simulink library "bipedlib"  (Simulink 6.1)
values from neighbouring files (symbols this model uses):
  D = [Db1, Db2, Db3, Db4 ... (first row only)    [pdparams.m]
  g = 9.81    [bipedparams.m]
  initstate =     [initstate.mat]
  l1 = 0.5    [bipedparams.m]    (also in pdparams.m = robot.l(2))
  l2 = 0.5    [bipedparams.m]    (also in pdparams.m = robot.l(3))
  P = [Pb1, Pb2, Pb3, Pb4 ... (first row only)    [pdparams.m]
  r0 = l0/2    (= 0.4)    [bipedparams.m]    (also in pdparams.m = robot.r(1))
  ref = [0.04, 0.3261, 0.0314, 0.2199]'    [pdparams.m]
  st = 0.005    [bipedparams.m]    (also in pdparams.m)
undefined symbols (not defined in the file or in its folder): dataprop, groundp, initswitch, knees, robot
libraries: bipedlib x11, simulink x6, crclib x1
(part 1 of 2)
settings Model: LastModifiedBy=Olli Haavisto

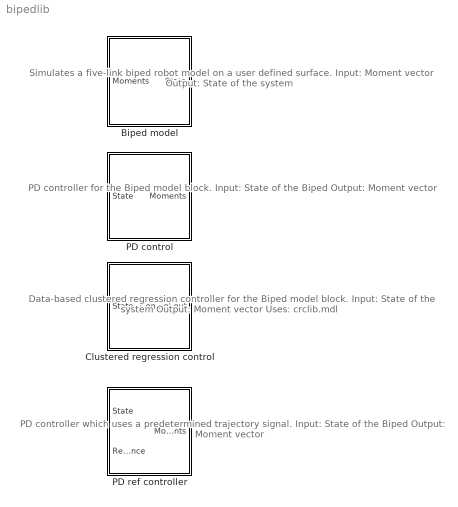
== system bipedlib ==
  note: Simulates a five-link biped robot model
      | on a user defined surface.
      | Input: Moment vector
      | Output: State of the system
  note: PD controller for the Biped model block.
      | Input: State of the Biped
      | Output: Moment vector
  note: Data-based clustered regression controller
      | for the Biped model block.
      | Input: State of the system
      | Output: Moment vector
      | Uses: crclib.mdl
  note: PD controller which uses a predetermined
      | trajectory signal.
      | Input: State of the Biped
      | Output: Moment vector
  Biped model : Subsystem  mask(Biped model){robot=robot, initstate=initstate, knees=knees, groundp=groundp, g=g, st=st}
      mask prompts: robot "Robot dimensions:"; initstate "Robot initial state:"; knees "Knee angle limiter parameters:"; groundp "Ground properties:"; g "Acceleration of gravity:"; st "Sample time:"
      mask help: The Biped model block simulates a 5-link biped walking robot on a user defined surface. The input is the moment vector and the output the state vector of the system.
      mask init:
      | % robot link lengths
      | l0 = robot.l(1); % torso
      | l1 = robot.l(2); % thigh
      | l2 = robot.l(3); % shank
      | % mass center locations
      | r0 = robot.r(1); % torso (from hip)
      | r1 = robot.r(2); % thigh (from hip)
      | r2 = robot.r(3); % shank (from knee)
      | % masses
      | m0 = robot.m(1); % torso
      | m1 = robot.m(2); % thigh
      | m2 = robot.m(3); % shank
      | % link inertias
      | J0 = robot.J(1);
      | J1 = robot.J(2);
      | J2 = robot.J(3);
      | 
      | % initial state
      | x00 = initstate.coordinates(1);
      | y00 = initstate.coordinates(2);
      | a0 = initstate.coordinates(3);
      | bl0 = initstate.coordinates(4);
      | br0 = initstate.coordinates(5);
      | cl0 = initstate.coordinates(6);
      | cr0 = initstate.coordinates(7);
      | 
      | % initial speeds
      | px00 = initstate.speeds(1);
      | py00 = initstate.speeds(2);
      | pa0 = initstate.speeds(3);
      | pbl0 = initstate.speeds(4);
      | pbr0 = initstate.speeds(5);
      | pcl0 = initstate.speeds(6);
      | pcr0 = initstate.speeds(7);
      | 
      | % initial ground contact state
      | gcstate = initstate.gcstate;
      | 
      | % knee angle limits
      | kneemin = knees.min;
      | kneemax = knees.max;
      | % knee stopper parameters
      | kk = knees.kk;
      | bk = knees.bk;
      | 
      | % ground shape
      | ground = groundp.ground;
      | % ground parameters
      | ky = groundp.ky;
      | by = groundp.by;
      | kx = groundp.kx;
      | bx = groundp.bx;
      | % friction coefficients
      | muk = groundp.muk; % kinetic
      | mus = groundp.mus; % static
      mask Display:
      | plot([0.0346, -0.0346, -0.0936, -0.2434],...
      |     [1.7739, 0.9769, 0.4804, 0.0034]);
      | plot([-0.0346, 0.0912, 0.1005],...
      |     [0.9769, 0.4930, -0.0069]);
      | plot([-0.5, 0.4], [0, 0]);
  Clustered regression control : Subsystem
  PD control : Subsystem
  PD ref controller : Subsystem

== system bipedlib/Biped model ==
  Moments : Inport  Port=1  LatchInput=off
  Dynamic model : Subsystem
  Ground contact : Subsystem  Orientation=left
  Knee stopper : Subsystem  Orientation=left
  Mux : Mux  Inputs=3
  Sum : Sum  Inputs=|++  SaturateOnIntegerOverflow=on
  To Workspace : ToWorkspace  VariableName=qout  SampleTime=-1  SaveFormat=Array
  To Workspace1 : ToWorkspace  VariableName=uout  SampleTime=st  SaveFormat=Array
  Zero-Order Hold : ZeroOrderHold  SampleTime=st
  Zero-Order Hold2 : ZeroOrderHold  SampleTime=st
  State : Outport
  wires:
  Dynamic model/1(q) -> Ground contact/1(q), Knee stopper/1(q), Mux/1
  Dynamic model/2(pq) -> Ground contact/2(pq), Knee stopper/2(pq), Mux/2
  Ground contact/1(Forces) -> Dynamic model/2(Forces)
  Knee stopper/1(Moments) -> Sum/2
  Moments/1 -> Zero-Order Hold2/1
  Sum/1 -> Dynamic model/1(Moments)
  Mux/1 -> Zero-Order Hold/1
  Zero-Order Hold/1 -> State/1, To Workspace/1
  Zero-Order Hold2/1 -> Sum/1, To Workspace1/1
  Ground contact/2(Sensors) -> Mux/3

== system bipedlib/Clustered regression control ==
  State : Inport  Port=1  PortDimensions=16  LatchInput=off
  Clustered regression : crclib/Clustered regression  pcrN=Nop  pcrpar=model  sigma2=sigma2  H1=H1
  Detect switch : Subsystem
  Postprocess : Subsystem
  Preprocess : Subsystem
  Saturation : Saturate  UpperLimit=50  LowerLimit=-50
  Switch controls : Subsystem
  Switch legs : Subsystem
  Control out : Outport
  wires:
  Preprocess/1(State out) -> Clustered regression/1
  State/1 -> Switch legs/1(State in), Detect switch/1(State)
  Switch legs/1(State out) -> Preprocess/1(State in)
  Clustered regression/1 -> Postprocess/1(Control in)
  Switch controls/1(Control out) -> Saturation/1
  Detect switch/1(Switch) -> Switch legs/2(Switch), Switch controls/2(Switch)
  Saturation/1 -> Control out/1
  Postprocess/1(Control out) -> Switch controls/1(Control in)

== system bipedlib/PD control ==
  State : Inport  Port=1  LatchInput=off
  Controller : Subsystem
  Create references : Subsystem
  Scope : Scope
      settings: SaveName=ScopeData3
  Selector : Selector  Elements=[1:7, 15, 16]  InputPortWidth=16
  Moments : Outport
  wires:
  Create references/1(Reference) -> Scope/1, Controller/2(Reference)
  State/1 -> Selector/1
  Controller/1(Moments) -> Moments/1
  Selector/1 -> Controller/1(State), Create references/1(State)

== system bipedlib/PD ref controller ==
  State : Inport  Port=1  LatchInput=off
  Reference : Inport  Port=2  LatchInput=off
  Convert to moments : Subsystem
  Detect phase : Subsystem
  Differences : Subsystem
  PDs : Subsystem
  Select parameters : Subsystem
  Selector : Selector  Elements=[1:7, 15, 16]  InputPortWidth=16
  Selector1 : Selector  Elements=[8,9]  InputPortWidth=9
  Smoothen : Subsystem
  Moments : Outport
  wires:
  Smoothen/1(Out) -> Moments/1
  Selector/1 -> Differences/1(State), Selector1/1
  PDs/1(Controls) -> Convert to moments/1(Controls)
  Differences/2(gamma_l) -> PDs/2(gamma_l)
  Convert to moments/1(moments) -> Smoothen/1(In)
  Differences/3(gamma_r) -> PDs/3(gamma_r)
  Differences/1(delta_beta) -> PDs/1(delta_beta)
  Differences/4(alpha) -> PDs/4(alpha)
  Select parameters/2(Ds) -> PDs/6(Ds)
  Detect phase/1(Phase number) -> Select parameters/1(Phase number)
  Select parameters/1(Ps) -> PDs/5(Ps)
  Selector1/1 -> Detect phase/1(Sensors)
  Reference/1 -> Differences/2(Reference)
  State/1 -> Selector/1

== system bipedlib/Biped model/Dynamic model ==
  Moments : Inport  Port=1  LatchInput=off
  Forces : Inport  Port=2  LatchInput=off
  A(q) : Subsystem  Orientation=left
  Integrator1 : Integrator  InitialCondition=[px00, py00, pa0, pbl0, pbr0, pcl0, pcr0]
  Integrator2 : Integrator  InitialCondition=[x00, y00, a0, bl0, br0, cl0, cr0]
  Inverse : Product  Orientation=left  Inputs=/  Multiplication=Matrix(*)  SaturateOnIntegerOverflow=on
  Mux : Mux  Orientation=left
  Product : Product  Orientation=left  Multiplication=Matrix(*)  SaturateOnIntegerOverflow=on
  "b(q, pq, M, F)" : Subsystem  Orientation=left
  q : Outport
  pq : Outport  Port=2
  wires:
  Integrator1/1 -> Integrator2/1, Mux/2, pq/1  "pq"
  Mux/1 -> "b(q, pq, M, F)"/1("q, pq, M, F")
  A(q)/1(A) -> Inverse/1
  Inverse/1 -> Product/1
  "b(q, pq, M, F)"/1(b) -> Product/2
  Product/1 -> Integrator1/1  "ppq"
  Moments/1 -> Mux/3
  Forces/1 -> Mux/4
  Integrator2/1 -> q/1, Mux/1, A(q)/1(q)  "q"

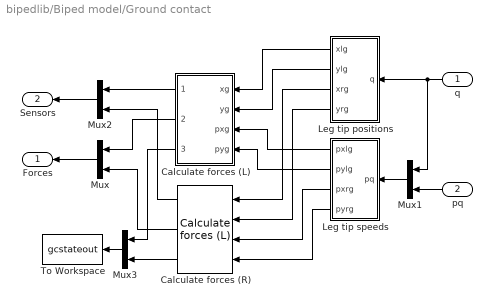
== system bipedlib/Biped model/Ground contact ==
  q : Inport  Orientation=left  Port=1  LatchInput=off
  pq : Inport  Orientation=left  Port=2  LatchInput=off
  Calculate forces (L) : Subsystem  Orientation=left  mask{gcstate=gcstate(1:2)}
  Calculate forces (R) : bipedlib/Biped model/Ground contact/Calculate forces (L)  Orientation=left  gcstate=gcstate(3:4)
  Leg tip positions : Subsystem  Orientation=left
  Leg tip speeds : Subsystem  Orientation=left
  Mux{,1..3} (4 alike) : Mux  Orientation=left  Inputs=2
  To Workspace : ToWorkspace  VariableName=gcstateout  SampleTime=st  SaveFormat=Array
  Forces : Outport  Orientation=left
  Sensors : Outport  Orientation=left  Port=2
  wires:
  pq/1 -> Mux1/2
  Mux1/1 -> Leg tip speeds/1(pq)
  q/1 -> Leg tip positions/1(q), Mux1/1
  Leg tip positions/3(xrg) -> Calculate forces (R)/1
  Leg tip positions/4(yrg) -> Calculate forces (R)/2
  Leg tip speeds/3(pxrg) -> Calculate forces (R)/3
  Leg tip speeds/4(pyrg) -> Calculate forces (R)/4
  Leg tip positions/1(xlg) -> Calculate forces (L)/1(xg)
  Leg tip positions/2(ylg) -> Calculate forces (L)/2(yg)
  Leg tip speeds/1(pxlg) -> Calculate forces (L)/3(pxg)
  Calculate forces (L)/2(Forces) -> Mux/1
  Mux/1 -> Forces/1
  Mux2/1 -> Sensors/1
  Calculate forces (L)/1(Sensor) -> Mux2/1
  Leg tip speeds/2(pylg) -> Calculate forces (L)/4(pyg)
  Calculate forces (L)/3(gcstate) -> Mux3/1
  Mux3/1 -> To Workspace/1
  Calculate forces (R)/1 -> Mux2/2
  Calculate forces (R)/2 -> Mux/2
  Calculate forces (R)/3 -> Mux3/2

== system bipedlib/Biped model/Knee stopper ==
  q : Inport  Orientation=left  Port=1  LatchInput=off
  pq : Inport  Orientation=left  Port=2  LatchInput=off
  Demux : Demux  Orientation=left  Outputs=2
  Demux1 : Demux  Orientation=left  Outputs=2
  Ground : Ground  Orientation=left
  Knee control (L) : Subsystem  Orientation=left
  Knee control (R) : bipedlib/Biped model/Knee stopper/Knee control (L)  Orientation=left  SimViewingDevice=off  DataTypeOverride=UseLocalSettings  MinMaxOverflowLogging=UseLocalSettings
      settings: Permissions=ReadWrite  RTWFcnNameOpts=Auto  RTWFileNameOpts=Auto
  Mux : Mux  Orientation=left
  Selector : Selector  Orientation=left  Elements=[6 7]  InputPortWidth=7
  Selector1 : Selector  Orientation=left  Elements=[6 7]  InputPortWidth=7
  Moments : Outport  Orientation=left
  wires:
  q/1 -> Selector/1
  Mux/1 -> Moments/1
  pq/1 -> Selector1/1
  Selector/1 -> Demux/1
  Selector1/1 -> Demux1/1
  Demux/1 -> Knee control (L)/1(Position)
  Demux/2 -> Knee control (R)/1
  Demux1/1 -> Knee control (L)/2(Speed)
  Demux1/2 -> Knee control (R)/2
  Knee control (L)/1(Moment) -> Mux/3
  Knee control (R)/1 -> Mux/4
  Ground/1 -> Mux/1, Mux/2

== system bipedlib/Clustered regression control/Detect switch ==
  State : Inport  Port=1  LatchInput=off
  Demux : Demux  Outputs=2
  Logical Operator1 : Logic  AllPortsSameDT=off
  Selector1 : Selector  Elements=[15, 16]  InputPortWidth=16
  Switch control : Subsystem  TreatAsAtomicUnit=on
  Switch : Outport
  wires:
  Switch control/1(Out1) -> Switch/1
  Demux/1 -> Logical Operator1/1
  Demux/2 -> Logical Operator1/2
  Selector1/1 -> Demux/1
  State/1 -> Selector1/1
  Logical Operator1/1 -> Switch control/Trigger

== system bipedlib/Clustered regression control/Postprocess ==
  Control in : Inport  Port=1  LatchInput=off
  Constant : Constant  Value=[dataprop.outputstd]
  Constant1 : Constant  Value=[dataprop.outputmean]
  Product : Product  Inputs=**  SaturateOnIntegerOverflow=on
  Sum : Sum  SaturateOnIntegerOverflow=on
  Control out : Outport
  wires:
  Constant/1 -> Product/2
  Constant1/1 -> Sum/2
  Control in/1 -> Product/1
  Product/1 -> Sum/1
  Sum/1 -> Control out/1

== system bipedlib/Clustered regression control/Preprocess ==
  State in : Inport  Port=1  LatchInput=off
  Constant : Constant  Value=[dataprop.inputstd, 1, 1]
  Constant1 : Constant  Value=[dataprop.inputmean, 0, 0]
  Product : Product  Inputs=*/  SaturateOnIntegerOverflow=on
  Selector2 : Selector  Elements=[2:16]  InputPortWidth=16
  Sum : Sum  Inputs=+-  SaturateOnIntegerOverflow=on
  State out : Outport
  wires:
  Constant1/1 -> Sum/2
  State in/1 -> Selector2/1
  Constant/1 -> Product/2
  Selector2/1 -> Sum/1
  Sum/1 -> Product/1
  Product/1 -> State out/1

== system bipedlib/Clustered regression control/Switch controls ==
  Control in : Inport  Port=1  LatchInput=off
  Switch : Inport  Port=2  PortDimensions=1  LatchInput=off
  Selector1 : Selector  Elements=[2, 1, 4, 3]  InputPortWidth=4
  Switch1 : Switch  Threshold=1  SaturateOnIntegerOverflow=on
  Control out : Outport
  wires:
  Switch1/1 -> Control out/1
  Control in/1 -> Switch1/1, Selector1/1
  Selector1/1 -> Switch1/3
  Switch/1 -> Switch1/2

== system bipedlib/Clustered regression control/Switch legs ==
  State in : Inport  Port=1  LatchInput=off
  Switch : Inport  Port=2  PortDimensions=1  LatchInput=off
  Selector : Selector  Elements=[1, 2, 3, 5, 4, 7, 6, 8, 9, 10, 12, 11, 14, 13, 16, 15]  InputPortWidth=16
  Switch1 : Switch  Threshold=1  SaturateOnIntegerOverflow=on
  State out : Outport
  wires:
  Switch/1 -> Switch1/2
  State in/1 -> Switch1/1, Selector/1
  Selector/1 -> Switch1/3
  Switch1/1 -> State out/1

== system bipedlib/PD control/Controller ==
  State : Inport  Port=1  LatchInput=off
  Reference : Inport  Port=2  LatchInput=off
  Convert to moments : Subsystem
  Detect phase : Subsystem
  Differences : Subsystem
  PDs : Subsystem
  Select parameters : Subsystem
  Selector1 : Selector  Elements=[8,9]  InputPortWidth=9
  Moments : Outport
  wires:
  State/1 -> Selector1/1, Differences/1(State)
  Reference/1 -> Differences/2(Reference)
  Selector1/1 -> Detect phase/1(Sensors)
  Select parameters/1(Ps) -> PDs/5(Ps)
  Detect phase/1(Phase number) -> Select parameters/1(Phase number), Convert to moments/2(phase)
  Select parameters/2(Ds) -> PDs/6(Ds)
  Differences/4(alpha) -> PDs/4(alpha)
  Differences/1(delta_beta) -> PDs/1(delta_beta)
  Differences/3(gamma_r) -> PDs/3(gamma_r)
  Convert to moments/1(moments) -> Moments/1
  Differences/2(gamma_l) -> PDs/2(gamma_l)
  PDs/1(Controls) -> Convert to moments/1(Controls)

== system bipedlib/PD control/Create references ==
  State : Inport  Port=1  LatchInput=off
  Saturation : Saturate  UpperLimit=[2*pi, 2*pi, pi, pi]  LowerLimit=[-2*pi, -2*pi, 0, 0]
  Store reference : UnitDelay  Orientation=left  X0=ref  SampleTime=st
  Switch references : Subsystem
  Walking cycle : Subsystem
  Reference : Outport
  wires:
  Walking cycle/1(New ref) -> Saturation/1
  Switch references/1(Out1) -> Reference/1
  Walking cycle/2(Switch) -> Switch references/2(Switch)
  State/1 -> Walking cycle/1(State)
  Saturation/1 -> Switch references/1(In1), Store reference/1
  Store reference/1 -> Walking cycle/2(Previous ref)

== system bipedlib/PD ref controller/Convert to moments ==
  Controls : Inport  Port=1  LatchInput=off
  Demux : Demux
  Gain : Gain  Gain=-1  SaturateOnIntegerOverflow=on
  Gain1 : Gain  Gain=0.5  SaturateOnIntegerOverflow=on
  Mux : Mux  Inputs=3
  Mux1 : Mux  Inputs=2
  Mux2 : Mux  Inputs=2
  Sum : Sum  SaturateOnIntegerOverflow=on
  moments : Outport
  wires:
  Sum/1 -> Mux/1
  Mux1/1 -> Sum/1
  Mux2/1 -> Sum/2
  Gain1/1 -> Mux2/2, Mux2/1
  Gain/1 -> Mux1/1
  Controls/1 -> Demux/1
  Demux/4 -> Gain1/1  "Control alpha"
  Demux/2 -> Mux/2  "Control gamma_l"
  Demux/3 -> Mux/3  "Control gamma_r"
  Mux/1 -> moments/1
  Demux/1 -> Mux1/2, Gain/1  "Control delta_beta"

== system bipedlib/PD ref controller/Detect phase ==
  note: 1: both legs on the ground
      | 2: left leg on the ground
      | 3: right leg on the ground
      | 4: neither of the legs on the ground
  Sensors : Inport  Port=1  LatchInput=off
  Constant4 : Constant  Value=[1, 2, 3, 4]
  Demux : Demux  Outputs=2
  Logical Operator{1,4..6} (4 alike) : Logic  AllPortsSameDT=off
  Logical Operator2 : Logic  Operator=NOT  AllPortsSameDT=off
  Logical Operator3 : Logic  Operator=NOT  AllPortsSameDT=off
  Mux : Mux
  Product4 : Product  SaturateOnIntegerOverflow=on
  Sum1 : Sum  Inputs=+  SaturateOnIntegerOverflow=on
  Phase number : Outport
  wires:
  Logical Operator6/1 -> Mux/4
  Logical Operator5/1 -> Mux/3
  Logical Operator4/1 -> Mux/2
  Logical Operator1/1 -> Mux/1
  Sum1/1 -> Phase number/1
  Product4/1 -> Sum1/1
  Mux/1 -> Product4/2
  Constant4/1 -> Product4/1
  Sensors/1 -> Demux/1
  Logical Operator2/1 -> Logical Operator6/2, Logical Operator5/1
  Logical Operator3/1 -> Logical Operator6/1, Logical Operator4/2
  Demux/2 -> Logical Operator5/2, Logical Operator3/1, Logical Operator1/2
  Demux/1 -> Logical Operator4/1, Logical Operator1/1, Logical Operator2/1

== system bipedlib/PD ref controller/Differences ==
  State : Inport  Port=1  LatchInput=off
  Reference : Inport  Port=2  LatchInput=off
  Demux1 : Demux
  Demux2 : Demux  Outputs=5
  Selector : Selector  Elements=[3:7]  InputPortWidth=9
  Sum1 : Sum  Inputs=+-+  SaturateOnIntegerOverflow=on
  Sum2 : Sum  Inputs=-+  SaturateOnIntegerOverflow=on
  Sum3 : Sum  Inputs=-+  SaturateOnIntegerOverflow=on
  Sum5 : Sum  Inputs=-+  SaturateOnIntegerOverflow=on
  delta_beta : Outport
  gamma_l : Outport  Port=2
  gamma_r : Outport  Port=3
  alpha : Outport  Port=4
  wires:
  Sum5/1 -> alpha/1
  Sum3/1 -> gamma_r/1
  Reference/1 -> Demux1/1
  Sum2/1 -> gamma_l/1
  Sum1/1 -> delta_beta/1
  State/1 -> Selector/1
  Demux1/4 -> Sum3/2  "gamma_r"
  Demux2/5 -> Sum3/1  "gamma_r"
  Demux1/3 -> Sum2/2  "gamma_l"
  Demux2/4 -> Sum2/1  "gamma_l"
  Demux1/2 -> Sum1/3  "delta_beta"
  Demux2/3 -> Sum1/2  "beta_r"
  Demux2/2 -> Sum1/1  "beta_l"
  Demux1/1 -> Sum5/2  "alpha"
  Demux2/1 -> Sum5/1  "alpha"
  Selector/1 -> Demux2/1

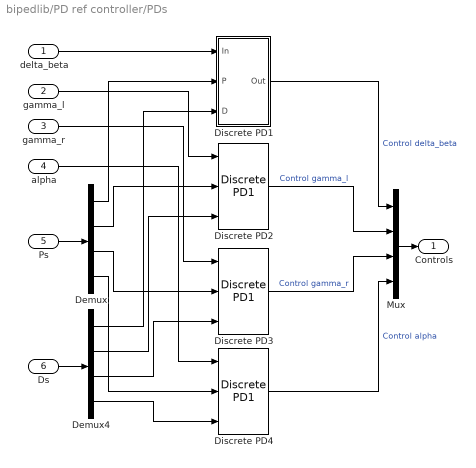
== system bipedlib/PD ref controller/PDs ==
  delta_beta : Inport  Port=1  LatchInput=off
  gamma_l : Inport  Port=2  LatchInput=off
  gamma_r : Inport  Port=3  LatchInput=off
  alpha : Inport  Port=4  LatchInput=off
  Ps : Inport  Port=5  LatchInput=off
  Ds : Inport  Port=6  LatchInput=off
  Demux : Demux
  Demux4 : Demux
  Discrete PD1 : Subsystem
  Discrete PD2 : bipedlib/PD ref controller/PDs/Discrete PD1
  Discrete PD3 : bipedlib/PD ref controller/PDs/Discrete PD1
  Discrete PD4 : bipedlib/PD ref controller/PDs/Discrete PD1
  Mux : Mux
  Controls : Outport
  wires:
  Mux/1 -> Controls/1
  Ds/1 -> Demux4/1
  Discrete PD4/1 -> Mux/4  "Control alpha"
  alpha/1 -> Discrete PD4/1
  Discrete PD3/1 -> Mux/3  "Control gamma_r"
  gamma_r/1 -> Discrete PD3/1
  Discrete PD2/1 -> Mux/2  "Control gamma_l"
  gamma_l/1 -> Discrete PD2/1
  Ps/1 -> Demux/1
  Discrete PD1/1(Out) -> Mux/1  "Control delta_beta"
  delta_beta/1 -> Discrete PD1/1(In)
  Demux4/4 -> Discrete PD4/3
  Demux4/3 -> Discrete PD3/3
  Demux4/2 -> Discrete PD2/3
  Demux4/1 -> Discrete PD1/3(D)
  Demux/4 -> Discrete PD4/2
  Demux/3 -> Discrete PD3/2
  Demux/2 -> Discrete PD2/2
  Demux/1 -> Discrete PD1/2(P)

== system bipedlib/PD ref controller/Select parameters ==
  Phase number : Inport  Port=1  LatchInput=off
  Constant : Constant  Value=P
  Constant2 : Constant  Value=D
  Selector2 : Selector  InputType=Matrix  Elements=[1 3]  Rows=-1  ColumnSrc=External  Columns=-1  InputPortWidth=3
  Selector4 : Selector  InputType=Matrix  Elements=[1 3]  Rows=-1  ColumnSrc=External  Columns=-1  InputPortWidth=3
  Ps : Outport
  Ds : Outport  Port=2
  wires:
  Phase number/1 -> Selector4/2, Selector2/2
  Selector4/1 -> Ds/1
  Selector2/1 -> Ps/1
  Constant2/1 -> Selector4/1
  Constant/1 -> Selector2/1

== system bipedlib/PD ref controller/Smoothen ==
  In : Inport  Port=1  LatchInput=off
  Demux : Demux
  Mux : Mux
  Weighted Moving Average{,1..3} (4 alike) : simulink/Discrete/Weighted Moving Average  mgainval=[0.2 0.4 0.3 0.1]  vinit=[0 0 0]  samptime=st  GainDataType=sfix( 16 )  MatRadixGroup=Best Precision: Matrix-wise  GainScaling=2^-10  OutDataType=sfix(16)  OutScaling=2^-10  DoSatur=off
  Out : Outport
  wires:
  Mux/1 -> Out/1
  Weighted Moving Average3/1 -> Mux/4
  Weighted Moving Average2/1 -> Mux/3
  Weighted Moving Average1/1 -> Mux/2
  Weighted Moving Average/1 -> Mux/1
  Demux/4 -> Weighted Moving Average3/1
  Demux/3 -> Weighted Moving Average2/1
  Demux/2 -> Weighted Moving Average1/1
  Demux/1 -> Weighted Moving Average/1
  In/1 -> Demux/1

== system bipedlib/Biped model/Dynamic model/A(q) ==
  q : Inport  Orientation=left  Port=1  LatchInput=off
  Matrix Concatenation : simulink/Math Operations/Matrix Concatenation  Orientation=left  numInports=7  catMethod=Horizontal
  column1 : Subsystem  Orientation=left
  column2 : Subsystem  Orientation=left
  column3 : Subsystem  Orientation=left
  column4 : Subsystem  Orientation=left
  column5 : Subsystem  Orientation=left
  column6 : Subsystem  Orientation=left
  column7 : Subsystem  Orientation=left
  A : Outport  Orientation=left
  wires:
  q/1 -> column1/1(In1), column2/1(In1), column3/1(In1), column4/1(In1), column7/1(In1), column6/1(In1), column5/1(In1)
  column1/1(Out1) -> Matrix Concatenation/1
  column2/1(Out1) -> Matrix Concatenation/2
  column3/1(Out1) -> Matrix Concatenation/3
  column4/1(Out1) -> Matrix Concatenation/4
  column6/1(Out1) -> Matrix Concatenation/6
  column5/1(Out1) -> Matrix Concatenation/5
  column7/1(Out1) -> Matrix Concatenation/7
  Matrix Concatenation/1 -> A/1

== system bipedlib/Biped model/Dynamic model/b(q, pq, M, F) ==
  "q, pq, M, F" : Inport  Orientation=left  Port=1  LatchInput=off
  Fcn : Fcn  Orientation=left  Expr=-(-u(19)-u(21)+2*m1*u(10)^2*r0*sin(u(3))+2*m2*u(10)^2*r0*sin(u(3))+l1*m2*u(10)^2*sin(u(3)-u(4))-2*l1*m2*u(10)*u(11)*sin(u(3)-u(4))+l1*m2*u(11)^2*sin(u(3)-u(4))+m1*u(10)^2*r1*sin(u(3)-u(4))-2*m1*u(10)*u(11)*r1*sin(u(3)-u(4))+m1*u(11)^2*r1*sin(u(3)-u(4))+l1*m2*u(10)^2*sin(u(3)-u(5))-2*l1*m2*u(10)*u(12)*sin(u(3)-u(5))+l1*m2*u(12)^2*sin(u(3)-u(5))+m1*u(10)^2*r1*sin(u(3)-u(5))-2*m1*u(10)*u(12)*r1*sin(u(3)-u(5))+m1*u(12)^2*r1*sin(u(3)-u(5))+m2*u(10)^2*r2*sin(u(3)-u(4)+u(6))-2*m2*u(10)*u(11)*r2*sin(u(3)-u(4)+u(6))+m2*u(11)^2*r2*sin(u(3)-u(4)+u(6))+2*m2*u(10)*u(13)*r2*sin(u(3)-u(4)+u(6))-2*m2*u(11)*u(13)*r2*sin(u(3)-u(4)+u(6))+m2*u(13)^2*r2*sin(u(3)-u(4)+u(6))+m2*u(10)^2*r2*sin(u(3)-u(5)+u(7))-2*m2*u(10)*u(12)*r2*sin(u(3)-u(5)+u(7))+m2*u(12)^2*r2*sin(u(3)-u(5)+u(7))+2*m2*u(10)*u(14)*r2*sin(u(3)-u(5)+u(7))-2*m2*u(12)*u(14)*r2*sin(u(3)-u(5)+u(7))+m2*u(14)^2*r2*sin(u(3)-u(5)+u(7)))
  Fcn1 : Fcn  Orientation=left  Expr=-(-u(20)-u(22)+g*m0+2.*g*m1+2.*g*m2+(2*m1+2.*m2)*u(10)^2*r0*cos(u(3))+(u(10)^2-2.*u(10)*u(11)+u(11)^2)*(l1*m2+m1*r1)*cos(u(3)-u(4))+l1*m2*u(10)^2*cos(u(3)-u(5))-2*l1*m2*u(10)*u(12)*cos(u(3)-u(5))+l1*m2*u(12)^2*cos(u(3)-u(5))+m1*u(10)^2*r1*cos(u(3)-u(5))-2*m1*u(10)*u(12)*r1*cos(u(3)-u(5))+m1*u(12)^2*r1*cos(u(3)-u(5))+m2*u(10)^2*r2*cos(u(3)-u(4)+u(6))-2*m2*u(10)*u(11)*r2*cos(u(3)-u(4)+u(6))+m2*u(11)^2*r2*cos(u(3)-u(4)+u(6))+2*m2*u(10)*u(13)*r2*cos(u(3)-u(4)+u(6))-2*m2*u(11)*u(13)*r2*cos(u(3)-u(4)+u(6))+m2*u(13)^2*r2*cos(u(3)-u(4)+u(6))+m2*u(10)^2*r2*cos(u(3)-u(5)+u(7))-2*m2*u(10)*u(12)*r2*cos(u(3)-u(5)+u(7))+m2*u(12)^2*r2*cos(u(3)-u(5)+u(7))+2*m2*u(10)*u(14)*r2*cos(u(3)-u(5)+u(7))-2*m2*u(12)*u(14)*r2*cos(u(3)-u(5)+u(7))+m2*u(14)^2*r2*cos(u(3)-u(5)+u(7)))
  Fcn2 : Fcn  Orientation=left  Expr=-((u(19)*r0+u(21)*r0)*cos(u(3))+u(19)*l1*cos(u(3)-u(4))+u(21)*l1*cos(u(3)-u(5))+u(19)*l2*cos(u(3)-u(4)+u(6))+u(21)*l2*cos(u(3)-u(5)+u(7))-u(20)*r0*sin(u(3))-u(22)*r0*sin(u(3))+2*g*m1*r0*sin(u(3))+2*g*m2*r0*sin(u(3))-u(20)*l1*sin(u(3)-u(4))+g*l1*m2*sin(u(3)-u(4))+g*m1*r1*sin(u(3)-u(4))-2*l1*m2*u(10)*u(11)*r0*sin(u(4))+l1*m2*u(11)^2*r0*sin(u(4))-2*m1*u(10)*u(11)*r0*r1*sin(u(4))+m1*u(11)^2*r0*r1*sin(u(4))-u(22)*l1*sin(u(3)-u(5))+g*l1*m2*sin(u(3)-u(5))+g*m1*r1*sin(u(3)-u(5))-2*l1*m2*u(10)*u(12)*r0*sin(u(5))+l1*m2*u(12)^2*r0*sin(u(5))-2*m1*u(10)*u(12)*r0*r1*sin(u(5))+m1*u(12)^2*r0*r1*sin(u(5))-2*m2*u(10)*u(11)*r0*r2*sin(u(4)-u(6))+m2*u(11)^2*r0*r2*sin(u(4)-u(6))+2*m2*u(10)*u(13)*r0*r2*sin(u(4)-u(6))-2*m2*u(11)*u(13)*r0*r2*sin(u(4)-u(6))+m2*u(13)^2*r0*r2*sin(u(4)-u(6))-2*l1*m2*u(10)*u(13)*r2*sin(u(6))+2*l1*m2*u(11)*u(13)*r2*sin(u(6))-l1*m2*u(13)^2*r2*sin(u(6))-u(20)*l2*sin(u(3)-u(4)+u(6))+g*m2*r2*sin(u(3)-u(4)+u(6))-2*m2*u(10)*u(12)*r0*r2*sin(u(5)-u(7))+m2*u(12)^2*r0*r2*sin(u(5)-u(7))+2*m2*u(10)*u(14)*r0*r2*sin(u(5)-u(7))-2*m2*u(12)*u(14)*r0*r2*sin(u(5)-u(7))+m2*u(14)^2*r0*r2*sin(u(5)-u(7))-2*l1*m2*u(10)*u(14)*r2*sin(u(7))+2*l1*m2*u(12)*u(14)*r2*sin(u(7))-l1*m2*u(14)^2*r2*sin(u(7))-u(22)*l2*sin(u(3)-u(5)+u(7))+g*m2*r2*sin(u(3)-u(5)+u(7)))
  Fcn3 : Fcn  Orientation=left  Expr=-(-u(15)-1.*u(19)*l1*cos(u(3)-u(4))-u(19)*l2*cos(u(3)-u(4)+u(6))+u(20)*l1*sin(u(3)-u(4))-g*l1*m2*sin(u(3)-u(4))-g*m1*r1*sin(u(3)-u(4))+l1*m2*u(10)^2*r0*sin(u(4))+m1*u(10)^2*r0*r1*sin(u(4))+m2*u(10)^2*r0*r2*sin(u(4)-u(6))+2*l1*m2*u(10)*u(13)*r2*sin(u(6))-2*l1*m2*u(11)*u(13)*r2*sin(u(6))+l1*m2*u(13)^2*r2*sin(u(6))+u(20)*l2*sin(u(3)-u(4)+u(6))-g*m2*r2*sin(u(3)-u(4)+u(6)))
  Fcn4 : Fcn  Orientation=left  Expr=-(-u(16)-1.*u(21)*l1*cos(u(3)-u(5))-u(21)*l2*cos(u(3)-u(5)+u(7))+u(22)*l1*sin(u(3)-u(5))-g*l1*m2*sin(u(3)-u(5))-g*m1*r1*sin(u(3)-u(5))+l1*m2*u(10)^2*r0*sin(u(5))+m1*u(10)^2*r0*r1*sin(u(5))+m2*u(10)^2*r0*r2*sin(u(5)-u(7))+2*l1*m2*u(10)*u(14)*r2*sin(u(7))-2*l1*m2*u(12)*u(14)*r2*sin(u(7))+l1*m2*u(14)^2*r2*sin(u(7))+u(22)*l2*sin(u(3)-u(5)+u(7))-g*m2*r2*sin(u(3)-u(5)+u(7)))
  Fcn5 : Fcn  Orientation=left  Expr=-(-u(17)+u(19)*l2*cos(u(3)-u(4)+u(6))-m2*u(10)^2*r0*r2*sin(u(4)-u(6))+l1*m2*u(10)^2*r2*sin(u(6))-2*l1*m2*u(10)*u(11)*r2*sin(u(6))+l1*m2*u(11)^2*r2*sin(u(6))-u(20)*l2*sin(u(3)-u(4)+u(6))+g*m2*r2*sin(u(3)-u(4)+u(6)))
  Fcn6 : Fcn  Orientation=left  Expr=-(-u(18)+u(21)*l2*cos(u(3)-u(5)+u(7))-m2*u(10)^2*r0*r2*sin(u(5)-u(7))+l1*m2*u(10)^2*r2*sin(u(7))-2*l1*m2*u(10)*u(12)*r2*sin(u(7))+l1*m2*u(12)^2*r2*sin(u(7))-u(22)*l2*sin(u(3)-u(5)+u(7))+g*m2*r2*sin(u(3)-u(5)+u(7)))
  Mux : Mux  Orientation=left  Inputs=7
  b : Outport  Orientation=left
  wires:
  "q, pq, M, F"/1 -> Fcn6/1, Fcn5/1, Fcn4/1, Fcn3/1, Fcn2/1, Fcn1/1, Fcn/1
  Fcn1/1 -> Mux/2
  Fcn2/1 -> Mux/3
  Fcn3/1 -> Mux/4
  Fcn4/1 -> Mux/5
  Fcn5/1 -> Mux/6
  Fcn6/1 -> Mux/7
  Mux/1 -> b/1
  Fcn/1 -> Mux/1

== system bipedlib/Biped model/Ground contact/Calculate forces (L) ==
  xg : Inport  Orientation=left  Port=1  LatchInput=off
  yg : Inport  Orientation=left  Port=2  LatchInput=off
  pxg : Inport  Orientation=left  Port=3  LatchInput=off
  pyg : Inport  Orientation=left  Port=4  LatchInput=off
  Controls : Subsystem  Orientation=left
  Data Type Conversion : DataTypeConversion  Orientation=left  OutDataTypeMode=double  SaturateOnIntegerOverflow=on  RndMeth=Zero
  Force projection : Subsystem  Orientation=left
  Leg tip projection : Subsystem  Orientation=left
  Sensor : Outport  Orientation=left
  Forces : Outport  Orientation=left  Port=2
  gcstate : Outport  Orientation=left  Port=3
  wires:
  Controls/1(Sensor) -> Data Type Conversion/1
  Leg tip projection/2(y'g) -> Controls/1(y'g)
  Leg tip projection/4(py'g) -> Controls/2(py'g)
  Leg tip projection/1(x'g) -> Controls/3(x'g)
  Leg tip projection/3(px'g) -> Controls/4(px'g)
  Controls/2(Forces) -> Force projection/1(F_t F_n)
  Leg tip projection/5(Ground vectors) -> Force projection/2(Ground vectors)
  xg/1 -> Leg tip projection/1(xg)
  yg/1 -> Leg tip projection/2(yg)
  Data Type Conversion/1 -> Sensor/1
  pxg/1 -> Leg tip projection/3(pxg)
  pyg/1 -> Leg tip projection/4(pyg)
  Force projection/1(Forces) -> Forces/1
  Controls/3(gcstate) -> gcstate/1

== system bipedlib/Biped model/Ground contact/Leg tip positions ==
  q : Inport  Orientation=down  Port=1  LatchInput=off
  Fcn : Fcn  Expr=u(1) - r0*sin(u(3)) - l1*sin(u(3)-u(4)) - l2*sin(u(3)-u(4)+u(6))
  Fcn1 : Fcn  Expr=u(2) - r0*cos(u(3)) - l1*cos(u(3)-u(4)) - l2*cos(u(3)-u(4)+u(6))
  Fcn2 : Fcn  Expr=u(1) - r0*sin(u(3)) - l1*sin(u(3)-u(5)) - l2*sin(u(3)-u(5)+u(7))
  Fcn3 : Fcn  Expr=u(2) - r0*cos(u(3)) - l1*cos(u(3)-u(5)) - l2*cos(u(3)-u(5)+u(7))
  xlg : Outport
  ylg : Outport  Port=2
  xrg : Outport  Port=3
  yrg : Outport  Port=4
  wires:
  q/1 -> Fcn/1, Fcn1/1, Fcn2/1, Fcn3/1
  Fcn/1 -> xlg/1
  Fcn1/1 -> ylg/1
  Fcn2/1 -> xrg/1
  Fcn3/1 -> yrg/1

== system bipedlib/Biped model/Ground contact/Leg tip speeds ==
  pq : Inport  Orientation=down  Port=1  LatchInput=off
  Fcn : Fcn  Expr=u(8) - r0*cos(u(3))*u(10) - l1*cos(u(3)-u(4))*(u(10)-u(11)) - l2*cos(u(3)-u(4)+u(6))*(u(10)-u(11)+u(13))
  Fcn1 : Fcn  Expr=u(8) - r0*cos(u(3))*u(10) - l1*cos(u(3)-u(5))*(u(10)-u(12)) - l2*cos(u(3)-u(5)+u(7))*(u(10)-u(12)+u(14))
  Fcn2 : Fcn  Expr=u(9) + r0*sin(u(3))*u(10) + l1*sin(u(3)-u(5))*(u(10)-u(12)) + l2*sin(u(3)-u(5)+u(7))*(u(10)-u(12)+u(14))
  Fcn3 : Fcn  Expr=u(9) + r0*sin(u(3))*u(10) + l1*sin(u(3)-u(4))*(u(10)-u(11)) + l2*sin(u(3)-u(4)+u(6))*(u(10)-u(11)+u(13))
  pxlg : Outport
  pylg : Outport  Port=2
  pxrg : Outport  Port=3
  pyrg : Outport  Port=4
  wires:
  Fcn2/1 -> pyrg/1
  Fcn1/1 -> pxrg/1
  Fcn3/1 -> pylg/1
  Fcn/1 -> pxlg/1
  pq/1 -> Fcn1/1, Fcn2/1, Fcn3/1, Fcn/1

== system bipedlib/Biped model/Knee stopper/Knee control (L) ==
  Position : Inport  Orientation=left  Port=1  LatchInput=off
  Speed : Inport  Orientation=left  Port=2  LatchInput=off
  Maximum angle limit : Constant  Orientation=left  Value=kneemax
  Minimum angle limit : Constant  Orientation=left  Value=kneemin
  PD : Subsystem  Orientation=left  TreatAsAtomicUnit=on
  PD1 : Subsystem  Orientation=left  TreatAsAtomicUnit=on
  Relational Operator : RelationalOperator  Orientation=left  Operator=<
  Relational Operator1 : RelationalOperator  Orientation=left  Operator=>
  Sum : Sum  Orientation=left  Inputs=|++  SaturateOnIntegerOverflow=on
  Moment : Outport  Orientation=left
  wires:
  Minimum angle limit/1 -> Relational Operator/2
  Position/1 -> Relational Operator/1, PD/1(Position), Relational Operator1/1, PD1/1(Position)
  Maximum angle limit/1 -> Relational Operator1/2
  Speed/1 -> PD/2(Speed), PD1/2(Speed)
  PD/1(Moment) -> Sum/1
  PD1/1(Moment) -> Sum/2
  Sum/1 -> Moment/1
  Relational Operator1/1 -> PD1/Enable
  Relational Operator/1 -> PD/Enable

== system bipedlib/Clustered regression control/Detect switch/Switch control ==
  note: 0 = right leg swings,
      | 1 = left leg swings
  Trigger : TriggerPort
  Logical Operator : Logic  Operator=NOT  AllPortsSameDT=off
  Store switch : UnitDelay  Orientation=left  X0=initswitch  SampleTime=-1
  Out1 : Outport  InitialOutput=initswitch
  wires:
  Store switch/1 -> Logical Operator/1
  Logical Operator/1 -> Out1/1, Store switch/1

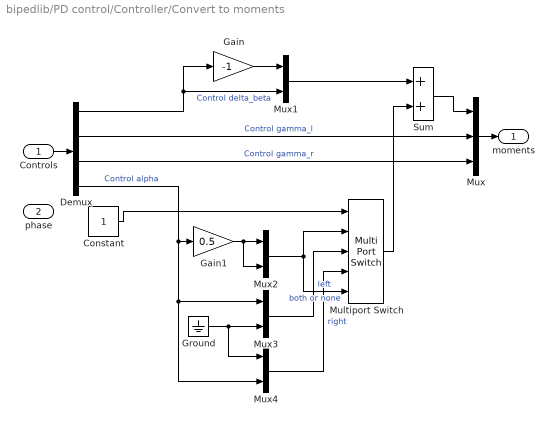
== system bipedlib/PD control/Controller/Convert to moments ==
  Controls : Inport  Port=1  LatchInput=off
  phase : Inport  Port=2  LatchInput=off
  Constant : Constant
  Demux : Demux
  Gain : Gain  Gain=-1  SaturateOnIntegerOverflow=on
  Gain1 : Gain  Gain=0.5  SaturateOnIntegerOverflow=on
  Ground : Ground
  Multiport Switch : MultiPortSwitch  SaturateOnIntegerOverflow=on
  Mux : Mux  Inputs=3
  Mux{1..4} (4 alike) : Mux  Inputs=2
  Sum : Sum  SaturateOnIntegerOverflow=on
  moments : Outport
  wires:
  Constant/1 -> Multiport Switch/1
  Demux/1 -> Gain/1, Mux1/2  "Control delta_beta"
  Mux/1 -> moments/1
  Demux/3 -> Mux/3  "Control gamma_r"
  Demux/2 -> Mux/2  "Control gamma_l"
  Demux/4 -> Gain1/1, Mux3/1, Mux4/2  "Control alpha"
  Controls/1 -> Demux/1
  Gain/1 -> Mux1/1
  Gain1/1 -> Mux2/1, Mux2/2
  Mux2/1 -> Multiport Switch/2, Multiport Switch/5  "both or none"
  Mux3/1 -> Multiport Switch/3  "left"
  Mux4/1 -> Multiport Switch/4  "right"
  Ground/1 -> Mux3/2, Mux4/1
  Multiport Switch/1 -> Sum/2
  Mux1/1 -> Sum/1
  Sum/1 -> Mux/1

== system bipedlib/PD control/Controller/Detect phase ==
  note: 1: both legs on the ground
      | 2: left leg on the ground
      | 3: right leg on the ground
      | 4: neither of the legs on the ground
  Sensors : Inport  Port=1  LatchInput=off
  Constant4 : Constant  Value=[1, 2, 3, 4]
  Demux : Demux  Outputs=2
  Logical Operator{1,4..6} (4 alike) : Logic  AllPortsSameDT=off
  Logical Operator2 : Logic  Operator=NOT  AllPortsSameDT=off
  Logical Operator3 : Logic  Operator=NOT  AllPortsSameDT=off
  Mux : Mux
  Product4 : Product  SaturateOnIntegerOverflow=on
  Sum1 : Sum  Inputs=+  SaturateOnIntegerOverflow=on
  Phase number : Outport
  wires:
  Demux/1 -> Logical Operator2/1, Logical Operator1/1, Logical Operator4/1
  Demux/2 -> Logical Operator1/2, Logical Operator3/1, Logical Operator5/2
  Logical Operator3/1 -> Logical Operator4/2, Logical Operator6/1
  Logical Operator2/1 -> Logical Operator5/1, Logical Operator6/2
  Sensors/1 -> Demux/1
  Constant4/1 -> Product4/1
  Mux/1 -> Product4/2
  Product4/1 -> Sum1/1
  Sum1/1 -> Phase number/1
  Logical Operator1/1 -> Mux/1
  Logical Operator4/1 -> Mux/2
  Logical Operator5/1 -> Mux/3
  Logical Operator6/1 -> Mux/4

== system bipedlib/PD control/Controller/Differences ==
  State : Inport  Port=1  LatchInput=off
  Reference : Inport  Port=2  LatchInput=off
  Demux1 : Demux
  Demux2 : Demux  Outputs=5
  Selector : Selector  Elements=[3:7]  InputPortWidth=9
  Sum1 : Sum  Inputs=+-+  SaturateOnIntegerOverflow=on
  Sum2 : Sum  Inputs=-+  SaturateOnIntegerOverflow=on
  Sum3 : Sum  Inputs=-+  SaturateOnIntegerOverflow=on
  Sum5 : Sum  Inputs=-+  SaturateOnIntegerOverflow=on
  delta_beta : Outport
  gamma_l : Outport  Port=2
  gamma_r : Outport  Port=3
  alpha : Outport  Port=4
  wires:
  Selector/1 -> Demux2/1
  Demux2/1 -> Sum5/1  "alpha"
  Demux1/1 -> Sum5/2  "alpha"
  Demux2/2 -> Sum1/1  "beta_l"
  Demux2/3 -> Sum1/2  "beta_r"
  Demux1/2 -> Sum1/3  "delta_beta"
  Demux2/4 -> Sum2/1  "gamma_l"
  Demux1/3 -> Sum2/2  "gamma_l"
  Demux2/5 -> Sum3/1  "gamma_r"
  Demux1/4 -> Sum3/2  "gamma_r"
  State/1 -> Selector/1
  Sum1/1 -> delta_beta/1
  Sum2/1 -> gamma_l/1
  Reference/1 -> Demux1/1
  Sum3/1 -> gamma_r/1
  Sum5/1 -> alpha/1

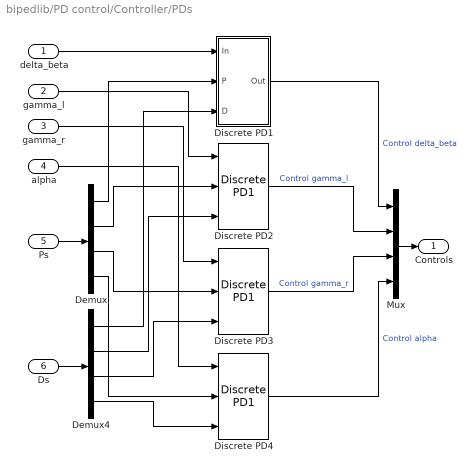
== system bipedlib/PD control/Controller/PDs ==
  delta_beta : Inport  Port=1  LatchInput=off
  gamma_l : Inport  Port=2  LatchInput=off
  gamma_r : Inport  Port=3  LatchInput=off
  alpha : Inport  Port=4  LatchInput=off
  Ps : Inport  Port=5  LatchInput=off
  Ds : Inport  Port=6  LatchInput=off
  Demux : Demux
  Demux4 : Demux
  Discrete PD1 : Subsystem
  Discrete PD2 : bipedlib/PD control/Controller/PDs/Discrete PD1
  Discrete PD3 : bipedlib/PD control/Controller/PDs/Discrete PD1
  Discrete PD4 : bipedlib/PD control/Controller/PDs/Discrete PD1
  Mux : Mux
  Controls : Outport
  wires:
  Demux/1 -> Discrete PD1/2(P)
  Demux/2 -> Discrete PD2/2
  Demux/3 -> Discrete PD3/2
  Demux/4 -> Discrete PD4/2
  Demux4/1 -> Discrete PD1/3(D)
  Demux4/2 -> Discrete PD2/3
  Demux4/3 -> Discrete PD3/3
  Demux4/4 -> Discrete PD4/3
  delta_beta/1 -> Discrete PD1/1(In)
  Discrete PD1/1(Out) -> Mux/1  "Control delta_beta"
  Ps/1 -> Demux/1
  gamma_l/1 -> Discrete PD2/1
  Discrete PD2/1 -> Mux/2  "Control gamma_l"
  gamma_r/1 -> Discrete PD3/1
  Discrete PD3/1 -> Mux/3  "Control gamma_r"
  alpha/1 -> Discrete PD4/1
  Discrete PD4/1 -> Mux/4  "Control alpha"
  Ds/1 -> Demux4/1
  Mux/1 -> Controls/1

== system bipedlib/PD control/Controller/Select parameters ==
  Phase number : Inport  Port=1  LatchInput=off
  Constant : Constant  Value=P
  Constant2 : Constant  Value=D
  Selector2 : Selector  InputType=Matrix  Elements=[1 3]  Rows=-1  ColumnSrc=External  Columns=-1  InputPortWidth=3
  Selector4 : Selector  InputType=Matrix  Elements=[1 3]  Rows=-1  ColumnSrc=External  Columns=-1  InputPortWidth=3
  Ps : Outport
  Ds : Outport  Port=2
  wires:
  Constant/1 -> Selector2/1
  Constant2/1 -> Selector4/1
  Selector2/1 -> Ps/1
  Selector4/1 -> Ds/1
  Phase number/1 -> Selector2/2, Selector4/2

== system bipedlib/PD control/Create references/Switch references ==
  In1 : Inport  Port=1  LatchInput=off
  Switch : Inport  Port=2  LatchInput=off
  Demux : Demux
  Gain : Gain  Gain=-1  SaturateOnIntegerOverflow=on
  Mux : Mux
  Switch1 : Switch  Threshold=1  SaturateOnIntegerOverflow=on
  Switch2 : Switch  Threshold=1  SaturateOnIntegerOverflow=on
  Switch3 : Switch  Threshold=1  SaturateOnIntegerOverflow=on
  Out1 : Outport
  wires:
  Mux/1 -> Out1/1
  Switch3/1 -> Mux/4
  Demux/4 -> Switch2/3, Switch3/1
  Demux/1 -> Mux/1
  Switch/1 -> Switch2/2, Switch1/2, Switch3/2
  In1/1 -> Demux/1
  Switch2/1 -> Mux/3
  Demux/3 -> Switch2/1, Switch3/3
  Switch1/1 -> Mux/2
  Demux/2 -> Switch1/1, Gain/1
  Gain/1 -> Switch1/3

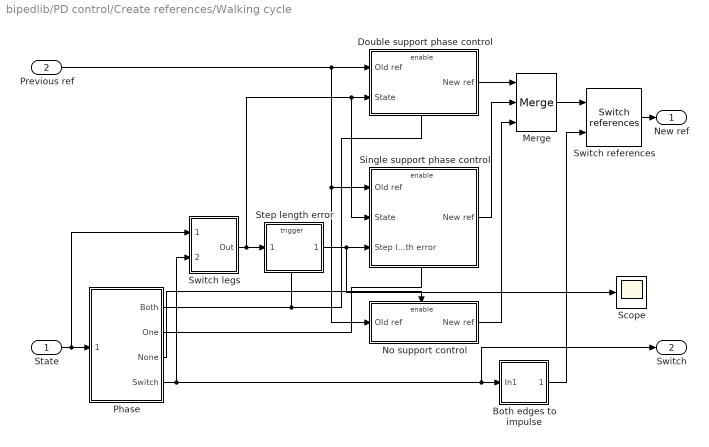
== system bipedlib/PD control/Create references/Walking cycle ==
  State : Inport  Port=1  LatchInput=off
  Previous ref : Inport  Port=2  LatchInput=off
  Both edges to impulse : Subsystem
  Double support phase control : Subsystem  TreatAsAtomicUnit=on
  Merge : Merge  Inputs=3
  No support control : Subsystem  TreatAsAtomicUnit=on
  Phase : Subsystem
  Scope : Scope
      settings: TimeRange=20  YMin=-0.04  YMax=0.06  SaveName=ScopeData2
  Single support phase control : Subsystem  TreatAsAtomicUnit=on
  Step length error : Subsystem
  Switch legs : Subsystem
  Switch references : bipedlib/PD control/Create references/Switch references
  New ref : Outport
  Switch : Outport  Port=2
  wires:
  Double support phase control/1(New ref) -> Merge/1
  Phase/2(One) -> Single support phase control/Enable
  Phase/3(None) -> No support control/Enable
  Single support phase control/1(New ref) -> Merge/2
  No support control/1(New ref) -> Merge/3
  Merge/1 -> Switch references/1
  Both edges to impulse/1(Out1) -> Switch references/2
  Switch references/1 -> New ref/1
  Previous ref/1 -> Single support phase control/1(Old ref), No support control/1(Old ref), Double support phase control/1(Old ref)
  Phase/1(Both) -> Double support phase control/Enable, Step length error/Trigger
  State/1 -> Phase/1(State in), Switch legs/1(State)
  Phase/4(Switch) -> Both edges to impulse/1(In1), Switch/1, Switch legs/2(Switch)
  Switch legs/1(Out) -> Step length error/1(State), Double support phase control/2(State), Single support phase control/2(State)
  Step length error/1(Error) -> Scope/1, Single support phase control/3(Step length error)

== system bipedlib/PD ref controller/PDs/Discrete PD1 ==
  In : Inport  Port=1  LatchInput=off
  P : Inport  Port=2  LatchInput=off
  D : Inport  Port=3  LatchInput=off
  Gain5 : Gain  Gain=1/st  SaturateOnIntegerOverflow=on
  Product : Product  SaturateOnIntegerOverflow=on
  Product1 : Product  Inputs=3  SaturateOnIntegerOverflow=on
  Relational Operator : RelationalOperator  Operator===
  Sum : Sum  SaturateOnIntegerOverflow=on
  Sum2 : Sum  Inputs=-+|  SaturateOnIntegerOverflow=on  InputSameDT=on
  Unit Delay : UnitDelay  SampleTime=-1
  Unit Delay2 : UnitDelay  SampleTime=-1
  Out : Outport
  wires:
  P/1 -> Product/1
  Relational Operator/1 -> Product1/3
  Unit Delay2/1 -> Relational Operator/2
  D/1 -> Relational Operator/1, Unit Delay2/1, Product1/2
  Product1/1 -> Gain5/1
  Sum2/1 -> Product1/1
  Sum/1 -> Out/1
  Gain5/1 -> Sum/2
  Unit Delay/1 -> Sum2/1
  In/1 -> Product/2, Unit Delay/1, Sum2/2
  Product/1 -> Sum/1

== system bipedlib/Biped model/Dynamic model/A(q)/column1 ==
  In1 : Inport  Orientation=left  Port=1  LatchInput=off
  Fcn : Fcn  Orientation=left  Expr=m0+2*m1+2*m2
  Fcn1 : Fcn  Orientation=left  Expr=0
  Fcn2 : Fcn  Orientation=left  Expr=(-2*m1*r0-2*m2*r0)*cos(u(3))+(-l1*m2-m1*r1)*cos(u(3)-u(4))-l1*m2*cos(u(3)-u(5))-m1*r1*cos(u(3)-u(5))-m2*r2*cos(u(3)-u(4)+u(6))-m2*r2*cos(u(3)-u(5)+u(7))
  Fcn3 : Fcn  Orientation=left  Expr=(l1*m2+m1*r1)*cos(u(3)-u(4))+m2*r2*cos(u(3)-u(4)+u(6))
  Fcn4 : Fcn  Orientation=left  Expr=(l1*m2+m1*r1)*cos(u(3)-u(5))+m2*r2*cos(u(3)-u(5)+u(7))
  Fcn5 : Fcn  Orientation=left  Expr=-m2*r2*cos(u(3)-u(4)+u(6))
  Fcn6 : Fcn  Orientation=left  Expr=-m2*r2*cos(u(3)-u(5)+u(7))
  Mux : Mux  Orientation=left  Inputs=7
  Out1 : Outport  Orientation=left
  wires:
  Mux/1 -> Out1/1
  In1/1 -> Fcn5/1, Fcn6/1, Fcn4/1, Fcn/1, Fcn1/1, Fcn2/1, Fcn3/1
  Fcn6/1 -> Mux/7
  Fcn5/1 -> Mux/6
  Fcn4/1 -> Mux/5
  Fcn3/1 -> Mux/4
  Fcn2/1 -> Mux/3
  Fcn1/1 -> Mux/2
  Fcn/1 -> Mux/1

== system bipedlib/Biped model/Dynamic model/A(q)/column2 ==
  In1 : Inport  Orientation=left  Port=1  LatchInput=off
  Fcn10 : Fcn  Orientation=left  Expr=(-l1*m2-m1*r1)*sin(u(3)-u(4))-m2*r2*sin(u(3)-u(4)+u(6))
  Fcn11 : Fcn  Orientation=left  Expr=(-l1*m2-m1*r1)*sin(u(3)-u(5))-m2*r2*sin(u(3)-u(5)+u(7))
  Fcn12 : Fcn  Orientation=left  Expr=m2*r2*sin(u(3)-u(4)+u(6))
  Fcn13 : Fcn  Orientation=left  Expr=m2*r2*sin(u(3)-u(5)+u(7))
  Fcn7 : Fcn  Orientation=left  Expr=0
  Fcn8 : Fcn  Orientation=left  Expr=m0+2*m1+2*m2
  Fcn9 : Fcn  Orientation=left  Expr=(2*m1*r0+2*m2*r0)*sin(u(3))+(l1*m2+m1*r1)*sin(u(3)-u(4))+l1*m2*sin(u(3)-u(5))+m1*r1*sin(u(3)-u(5))+m2*r2*sin(u(3)-u(4)+u(6))+m2*r2*sin(u(3)-u(5)+u(7))
  Mux : Mux  Orientation=left  Inputs=7
  Out1 : Outport  Orientation=left
  wires:
  Fcn7/1 -> Mux/1
  Fcn8/1 -> Mux/2
  Fcn9/1 -> Mux/3
  Fcn10/1 -> Mux/4
  Fcn11/1 -> Mux/5
  Fcn12/1 -> Mux/6
  Fcn13/1 -> Mux/7
  In1/1 -> Fcn8/1, Fcn7/1, Fcn9/1, Fcn13/1, Fcn12/1, Fcn11/1, Fcn10/1
  Mux/1 -> Out1/1

== system bipedlib/Biped model/Dynamic model/A(q)/column3 ==
  In1 : Inport  Orientation=left  Port=1  LatchInput=off
  Fcn14 : Fcn  Orientation=left  Expr=-J1-J2-l1^2*m2-m1*r1^2-m2*r2^2+(-l1*m2*r0-m1*r0*r1)*cos(u(4))-m2*r0*r2*cos(u(4)-u(6))-2*l1*m2*r2*cos(u(6))
  Fcn15 : Fcn  Orientation=left  Expr=-J1-J2-l1^2*m2-m1*r1^2-m2*r2^2+(-l1*m2*r0-m1*r0*r1)*cos(u(5))-m2*r0*r2*cos(u(5)-u(7))-2*l1*m2*r2*cos(u(7))
  Fcn16 : Fcn  Orientation=left  Expr=J2+m2*r2^2+m2*r0*r2*cos(u(4)-u(6))+l1*m2*r2*cos(u(6))
  Fcn17 : Fcn  Orientation=left  Expr=J2+m2*r2^2+m2*r0*r2*cos(u(5)-u(7))+l1*m2*r2*cos(u(7))
  Fcn18 : Fcn  Orientation=left  Expr=(-2*m1*r0-2*m2*r0)*cos(u(3))+(-l1*m2-m1*r1)*cos(u(3)-u(4))-l1*m2*cos(u(3)-u(5))-m1*r1*cos(u(3)-u(5))-m2*r2*cos(u(3)-u(4)+u(6))-m2*r2*cos(u(3)-u(5)+u(7))
  Fcn19 : Fcn  Orientation=left  Expr=(2*m1*r0+2*m2*r0)*sin(u(3))+(l1*m2+m1*r1)*sin(u(3)-u(4))+l1*m2*sin(u(3)-u(5))+m1*r1*sin(u(3)-u(5))+m2*r2*sin(u(3)-u(4)+u(6))+m2*r2*sin(u(3)-u(5)+u(7))
  Fcn20 : Fcn  Orientation=left  Expr=J0+2*J1+2*J2+2*l1^2*m2+2*m1*r0^2+2*m2*r0^2+2*m1*r1^2+2*m2*r2^2+(2*l1*m2*r0+2*m1*r0*r1)*cos(u(4))+(2*l1*m2*r0+2*m1*r0*r1)*cos(u(5))+2*m2*r0*r2*cos(u(4)-u(6))+2*l1*m2*r2*cos(u(6))+2*m2*r0*r2*cos(u(5)-u(7))+2*l1*m2*r2*cos(u(7))
  Mux : Mux  Orientation=left  Inputs=7
  Out1 : Outport  Orientation=left
  wires:
  Mux/1 -> Out1/1
  In1/1 -> Fcn16/1, Fcn17/1, Fcn15/1, Fcn18/1, Fcn19/1, Fcn20/1, Fcn14/1
  Fcn17/1 -> Mux/7
  Fcn16/1 -> Mux/6
  Fcn15/1 -> Mux/5
  Fcn14/1 -> Mux/4
  Fcn20/1 -> Mux/3
  Fcn19/1 -> Mux/2
  Fcn18/1 -> Mux/1

== system bipedlib/Biped model/Dynamic model/A(q)/column4 ==
  In1 : Inport  Orientation=left  Port=1  LatchInput=off
  Fcn21 : Fcn  Orientation=left  Expr=J1+J2+l1^2*m2+m1*r1^2+m2*r2^2+2*l1*m2*r2*cos(u(6))
  Fcn22 : Fcn  Orientation=left  Expr=0
  Fcn23 : Fcn  Orientation=left  Expr=-J2-m2*r2^2-l1*m2*r2*cos(u(6))
  Fcn24 : Fcn  Orientation=left  Expr=0
  Fcn25 : Fcn  Orientation=left  Expr=(l1*m2+m1*r1)*cos(u(3)-u(4))+m2*r2*cos(u(3)-u(4)+u(6))
  Fcn26 : Fcn  Orientation=left  Expr=(-l1*m2-m1*r1)*sin(u(3)-u(4))-m2*r2*sin(u(3)-u(4)+u(6))
  Fcn27 : Fcn  Orientation=left  Expr=-J1-J2-l1^2*m2-m1*r1^2-m2*r2^2+r0*(-l1*m2-m1*r1)*cos(u(4))-m2*r0*r2*cos(u(4)-u(6))-2*l1*m2*r2*cos(u(6))
  Mux : Mux  Orientation=left  Inputs=7
  Out1 : Outport  Orientation=left
  wires:
  Fcn25/1 -> Mux/1
  Fcn26/1 -> Mux/2
  Fcn27/1 -> Mux/3
  Fcn21/1 -> Mux/4
  Fcn22/1 -> Mux/5
  Fcn23/1 -> Mux/6
  Fcn24/1 -> Mux/7
  In1/1 -> Fcn26/1, Fcn25/1, Fcn27/1, Fcn24/1, Fcn23/1, Fcn22/1, Fcn21/1
  Mux/1 -> Out1/1

== system bipedlib/Biped model/Dynamic model/A(q)/column5 ==
  In1 : Inport  Orientation=left  Port=1  LatchInput=off
  Fcn28 : Fcn  Orientation=left  Expr=0
  Fcn29 : Fcn  Orientation=left  Expr=J1+J2+l1^2*m2+m1*r1^2+m2*r2^2+2*l1*m2*r2*cos(u(7))
  Fcn30 : Fcn  Orientation=left  Expr=0
  Fcn31 : Fcn  Orientation=left  Expr=-J2-m2*r2^2-l1*m2*r2*cos(u(7))
  Fcn32 : Fcn  Orientation=left  Expr=(l1*m2+m1*r1)*cos(u(3)-u(5))+m2*r2*cos(u(3)-u(5)+u(7))
  Fcn33 : Fcn  Orientation=left  Expr=(-l1*m2-m1*r1)*sin(u(3)-u(5))-m2*r2*sin(u(3)-u(5)+u(7))
  Fcn34 : Fcn  Orientation=left  Expr=-J1-J2-l1^2*m2-m1*r1^2-m2*r2^2+r0*(-l1*m2-m1*r1)*cos(u(5))-m2*r0*r2*cos(u(5)-u(7))-2*l1*m2*r2*cos(u(7))
  Mux : Mux  Orientation=left  Inputs=7
  Out1 : Outport  Orientation=left
  wires:
  Mux/1 -> Out1/1
  In1/1 -> Fcn30/1, Fcn31/1, Fcn29/1, Fcn32/1, Fcn33/1, Fcn34/1, Fcn28/1
  Fcn31/1 -> Mux/7
  Fcn30/1 -> Mux/6
  Fcn29/1 -> Mux/5
  Fcn28/1 -> Mux/4
  Fcn34/1 -> Mux/3
  Fcn33/1 -> Mux/2
  Fcn32/1 -> Mux/1

== system bipedlib/Biped model/Dynamic model/A(q)/column6 ==
  In1 : Inport  Orientation=left  Port=1  LatchInput=off
  Fcn35 : Fcn  Orientation=left  Expr=-J2-m2*r2^2-l1*m2*r2*cos(u(6))
  Fcn36 : Fcn  Orientation=left  Expr=0
  Fcn37 : Fcn  Orientation=left  Expr=J2+m2*r2^2
  Fcn38 : Fcn  Orientation=left  Expr=0
  Fcn39 : Fcn  Orientation=left  Expr=-m2*r2*cos(u(3)-u(4)+u(6))
  Fcn40 : Fcn  Orientation=left  Expr=m2*r2*sin(u(3)-u(4)+u(6))
  Fcn41 : Fcn  Orientation=left  Expr=J2+m2*r2^2+m2*r0*r2*cos(u(4)-u(6))+l1*m2*r2*cos(u(6))
  Mux : Mux  Orientation=left  Inputs=7
  Out1 : Outport  Orientation=left
  wires:
  Fcn39/1 -> Mux/1
  Fcn40/1 -> Mux/2
  Fcn41/1 -> Mux/3
  Fcn35/1 -> Mux/4
  Fcn36/1 -> Mux/5
  Fcn37/1 -> Mux/6
  Fcn38/1 -> Mux/7
  In1/1 -> Fcn40/1, Fcn39/1, Fcn41/1, Fcn38/1, Fcn37/1, Fcn36/1, Fcn35/1
  Mux/1 -> Out1/1

== system bipedlib/Biped model/Dynamic model/A(q)/column7 ==
  In1 : Inport  Orientation=left  Port=1  LatchInput=off
  Fcn42 : Fcn  Orientation=left  Expr=0
  Fcn43 : Fcn  Orientation=left  Expr=-J2-m2*r2^2-l1*m2*r2*cos(u(7))
  Fcn44 : Fcn  Orientation=left  Expr=0
  Fcn45 : Fcn  Orientation=left  Expr=J2+m2*r2^2
  Fcn46 : Fcn  Orientation=left  Expr=-m2*r2*cos(u(3)-u(5)+u(7))
  Fcn47 : Fcn  Orientation=left  Expr=m2*r2*sin(u(3)-u(5)+u(7))
  Fcn48 : Fcn  Orientation=left  Expr=J2+m2*r2^2+m2*r0*r2*cos(u(5)-u(7))+l1*m2*r2*cos(u(7))
  Mux : Mux  Orientation=left  Inputs=7
  Out1 : Outport  Orientation=left
  wires:
  Fcn46/1 -> Mux/1
  Fcn47/1 -> Mux/2
  Fcn48/1 -> Mux/3
  Fcn42/1 -> Mux/4
  Fcn43/1 -> Mux/5
  Fcn44/1 -> Mux/6
  Fcn45/1 -> Mux/7
  In1/1 -> Fcn42/1, Fcn46/1, Fcn47/1, Fcn48/1, Fcn43/1, Fcn44/1, Fcn45/1
  Mux/1 -> Out1/1

== system bipedlib/Biped model/Ground contact/Calculate forces (L)/Controls ==
  y'g : Inport  Orientation=left  Port=1  LatchInput=off
  py'g : Inport  Orientation=left  Port=2  LatchInput=off
  x'g : Inport  Orientation=left  Port=3  LatchInput=off
  px'g : Inport  Orientation=left  Port=4  LatchInput=off
  Control x'g : Subsystem  Orientation=left
  Control y'g : Subsystem  Orientation=left
  Mux1 : Mux  Orientation=left  Inputs=2
  Sensor : Outport  Orientation=left
  Forces : Outport  Orientation=left  Port=2
  gcstate : Outport  Orientation=left  Port=3
  wires:
  Control y'g/1(Force) -> Mux1/2, Control x'g/4(Normal force)
  Control y'g/2(Sensor) -> Control x'g/1(Sensor), Sensor/1
  y'g/1 -> Control y'g/1(Position)
  py'g/1 -> Control y'g/2(Speed)
  x'g/1 -> Control x'g/2(Position)
  px'g/1 -> Control x'g/3(Speed)
  Control x'g/1(Force) -> Mux1/1
  Mux1/1 -> Forces/1
  Control x'g/2(gcstate) -> gcstate/1

== system bipedlib/Biped model/Ground contact/Calculate forces (L)/Force projection ==
  F_t F_n : Inport  Orientation=left  Port=1  LatchInput=off
  Ground vectors : Inport  Orientation=left  Port=2  LatchInput=off
  Demux : Demux  Orientation=left  Outputs=2
  Demux1 : Demux  Orientation=left  Outputs=2
  Product : Product  Orientation=left  SaturateOnIntegerOverflow=on
  Product1 : Product  Orientation=left  SaturateOnIntegerOverflow=on
  Sum : Sum  Orientation=left  SaturateOnIntegerOverflow=on
  Forces : Outport  Orientation=left
  wires:
  Demux1/1 -> Product/2
  F_t F_n/1 -> Demux/1
  Demux/1 -> Product/1
  Demux/2 -> Product1/1
  Demux1/2 -> Product1/2
  Product1/1 -> Sum/2
  Product/1 -> Sum/1
  Sum/1 -> Forces/1
  Ground vectors/1 -> Demux1/1

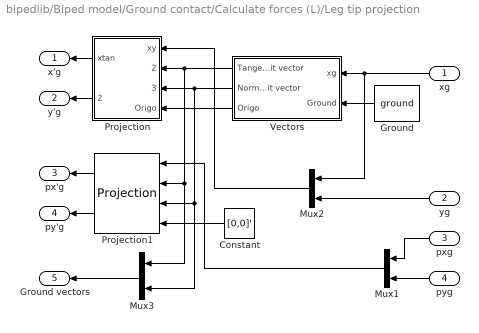
== system bipedlib/Biped model/Ground contact/Calculate forces (L)/Leg tip projection ==
  xg : Inport  Orientation=left  Port=1  LatchInput=off
  yg : Inport  Orientation=left  Port=2  LatchInput=off
  pxg : Inport  Orientation=left  Port=3  LatchInput=off
  pyg : Inport  Orientation=left  Port=4  LatchInput=off
  Constant : Constant  Orientation=left  Value=[0,0]'  VectorParams1D=off
  Ground : Constant  Orientation=left  Value=ground
  Mux1 : Mux  Orientation=left  Inputs=2
  Mux2 : Mux  Orientation=left  Inputs=2
  Mux3 : Mux  Orientation=left  Inputs=2
  Projection : Subsystem  Orientation=left
  Projection1 : bipedlib/Biped model/Ground contact/Calculate forces (L)/Leg tip projection/Projection  Orientation=left  SimViewingDevice=off  DataTypeOverride=UseLocalSettings  MinMaxOverflowLogging=UseLocalSettings
      settings: Permissions=ReadWrite  RTWFcnNameOpts=Auto  RTWFileNameOpts=Auto
  Vectors : Subsystem  Orientation=left
  x'g : Outport  Orientation=left
  y'g : Outport  Orientation=left  Port=2
  px'g : Outport  Orientation=left  Port=3
  py'g : Outport  Orientation=left  Port=4
  Ground vectors : Outport  Orientation=left  Port=5
  wires:
  Projection/2(ynorm) -> y'g/1
  Projection/1(xtan) -> x'g/1
  pxg/1 -> Mux1/1
  pyg/1 -> Mux1/2
  Mux1/1 -> Projection1/1
  Projection1/1 -> px'g/1
  Projection1/2 -> py'g/1
  Ground/1 -> Vectors/2(Ground)
  xg/1 -> Vectors/1(xg), Mux2/1
  Vectors/3(Origo) -> Projection/4(Origo)
  Vectors/2(Normal unit vector) -> Projection/3(Normal), Mux3/2, Projection1/3
  Vectors/1(Tangential unit vector) -> Projection/2(Tangential), Mux3/1, Projection1/2
  Mux2/1 -> Projection/1(xy)
  yg/1 -> Mux2/2
  Constant/1 -> Projection1/4
  Mux3/1 -> Ground vectors/1
